simulink model "SPContinuousSimulink"  (R2023b)
settings: Solver=VariableStepAuto  StartTime=0.0  StopTime=Tsim  RelTol=1e-3
values from neighbouring files (symbols this model uses):
  denp = [3 1]    [SPContinuous.m]
  h = 6.5    [SPContinuous.m]
  nump = 2    [SPContinuous.m]
libraries: cstblocks x4
settings Model: Creator=klysm  LastModifiedBy=klysm

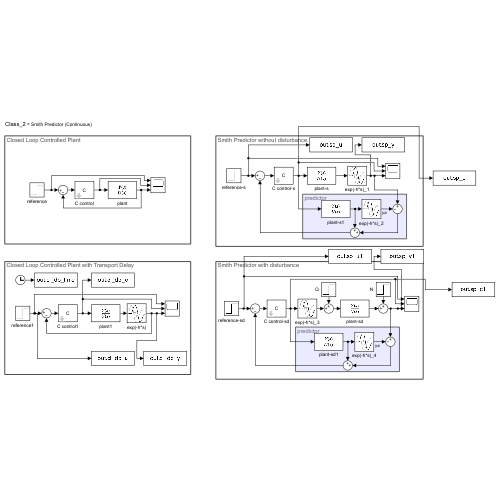
[thumbnail: Simulink's stored preview of the top-level diagram]
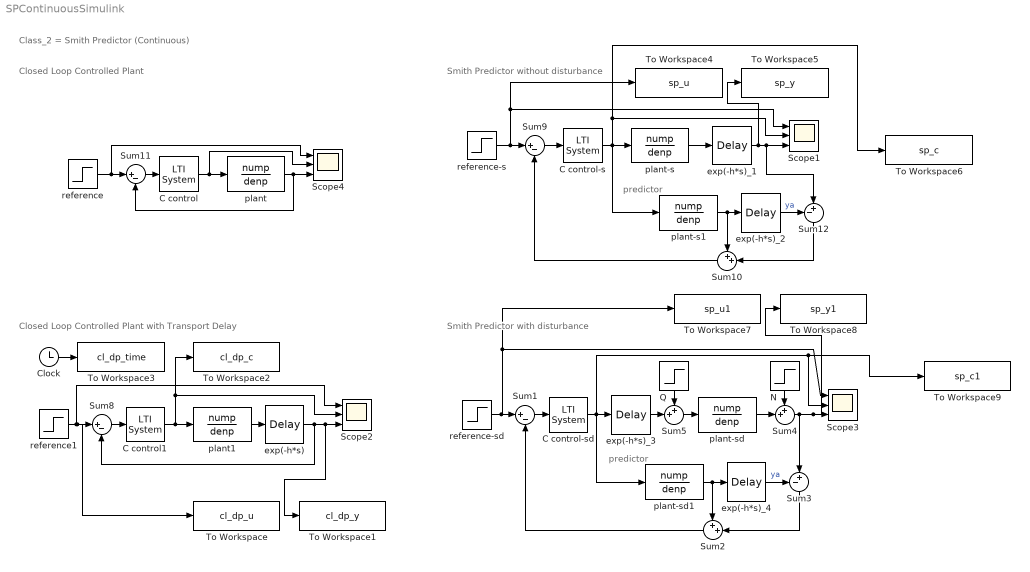
== system SPContinuousSimulink ==
  note: Class_2 = Smith Predictor (Continuous)
  note: Smith Predictor without disturbance
  note: predictor
  note: Smith Predictor with disturbance
  note: Closed Loop Controlled Plant with Transport Delay
  note: Closed Loop Controlled Plant
  note: predictor
  C control : cstblocks/LTI System  sys=C  IC=[]  PadeOrder=0
  C control-s : cstblocks/LTI System  sys=C  IC=[]  PadeOrder=0
  C control-sd : cstblocks/LTI System  sys=C  IC=[]  PadeOrder=0
  C control1 : cstblocks/LTI System  sys=C  IC=[]  PadeOrder=0
  Clock : Clock
  N : Step  Time=20  After=0.2  SampleTime=0
  Q : Step  Time=10  After=0.2  SampleTime=0
  Scope{1..4} (4 alike) : Scope  NumInputPorts=3
  Sum{1,8..9,11} (4 alike) : Sum  Inputs=|+-
  Sum{2,4..5,10} (4 alike) : Sum  Inputs=++|
  Sum12 : Sum  Inputs=-+|
  Sum3 : Sum  Inputs=-+|
  To Workspace : ToWorkspace  VariableName=cl_dp_u  SampleTime=-1
  To Workspace1 : ToWorkspace  VariableName=cl_dp_y  SampleTime=-1
  To Workspace2 : ToWorkspace  VariableName=cl_dp_c  SampleTime=-1
  To Workspace3 : ToWorkspace  VariableName=cl_dp_time  SampleTime=-1
  To Workspace4 : ToWorkspace  VariableName=sp_u  SampleTime=-1
  To Workspace5 : ToWorkspace  VariableName=sp_y  SampleTime=-1
  To Workspace6 : ToWorkspace  VariableName=sp_c  SampleTime=-1
  To Workspace7 : ToWorkspace  VariableName=sp_u1  SampleTime=-1
  To Workspace8 : ToWorkspace  VariableName=sp_y1  SampleTime=-1
  To Workspace9 : ToWorkspace  VariableName=sp_c1  SampleTime=-1
  exp(-h*s) : TransportDelay
  exp(-h*s)_{1..4} (4 alike) : TransportDelay  DelayTime=h
  plant : TransferFcn  Numerator=nump  Denominator=denp
  plant-s : TransferFcn  Numerator=nump  Denominator=denp
  plant-s1 : TransferFcn  Numerator=nump  Denominator=denp
  plant-sd : TransferFcn  Numerator=nump  Denominator=denp
  plant-sd1 : TransferFcn  Numerator=nump  Denominator=denp
  plant1 : TransferFcn  Numerator=nump  Denominator=denp
  reference : Step  Time=0  SampleTime=0
  reference-s : Step  Time=0  SampleTime=0
  reference-sd : Step  Time=0  SampleTime=0
  reference1 : Step  Time=0  SampleTime=0
  wires:
  reference-sd/1 -> To Workspace7/1, Scope3/1, Sum1/1
  Sum1/1 -> C control-sd/1
  exp(-h*s)_4/1 -> Sum3/1  "ya"
  C control-sd/1 -> plant-sd1/1, exp(-h*s)_3/1, To Workspace9/1, Scope3/2
  Sum3/1 -> Sum2/2
  Sum2/1 -> Sum1/2
  plant-sd1/1 -> Sum2/1, exp(-h*s)_4/1
  C control/1 -> Scope4/2, plant/1
  Sum11/1 -> C control/1
  reference/1 -> Scope4/1, Sum11/1
  plant/1 -> Scope4/3, Sum11/2
  reference1/1 -> To Workspace/1, Sum8/1, Scope2/1
  Sum8/1 -> C control1/1
  C control1/1 -> To Workspace2/1, Scope2/2, plant1/1
  plant1/1 -> exp(-h*s)/1
  exp(-h*s)/1 -> To Workspace1/1, Scope2/3, Sum8/2
  N/1 -> Sum4/1
  plant-sd/1 -> Sum4/2
  Sum4/1 -> To Workspace8/1, Scope3/3, Sum3/2
  C control-s/1 -> To Workspace6/1, Scope1/2, plant-s/1, plant-s1/1
  exp(-h*s)_2/1 -> Sum12/1  "ya"
  exp(-h*s)_1/1 -> Scope1/3, Sum12/2, To Workspace5/1
  plant-s/1 -> exp(-h*s)_1/1
  plant-s1/1 -> Sum10/1, exp(-h*s)_2/1
  Sum12/1 -> Sum10/2
  Sum9/1 -> C control-s/1
  Sum10/1 -> Sum9/2
  reference-s/1 -> To Workspace4/1, Scope1/1, Sum9/1
  Sum5/1 -> plant-sd/1
  Q/1 -> Sum5/1
  Clock/1 -> To Workspace3/1
  exp(-h*s)_3/1 -> Sum5/2
